simulink model "Immersion_2"  (Simulink 9.1)
settings: Solver=ode45  StartTime=0.0  StopTime=6  FixedStep=0.01  RelTol=1e-3  EnableMultiTasking=on
model workspace (MAT data in the model file):
  random_seed : num (value not decoded)
undefined symbols (not defined in the file): CafHat, CarHat, K, lam_1, lam_2, Lf, Lr, m, mu, random_seeds, Vel
libraries: simulink x2, Solver_SF x1
settings Model: Creator=xuwei  LastModifiedBy=CK12
settings DataIOCC: LimitDataPoints=on
settings OptimizationCC: ExpressionDepthLimit=2147483647
settings DebuggingCC: SolverPrmCheckMsg=warning  FcnCallInpInsideContextMsg=warning  StateNameClashWarn=warning
settings ConfigComp: CovHtmlReporting=off

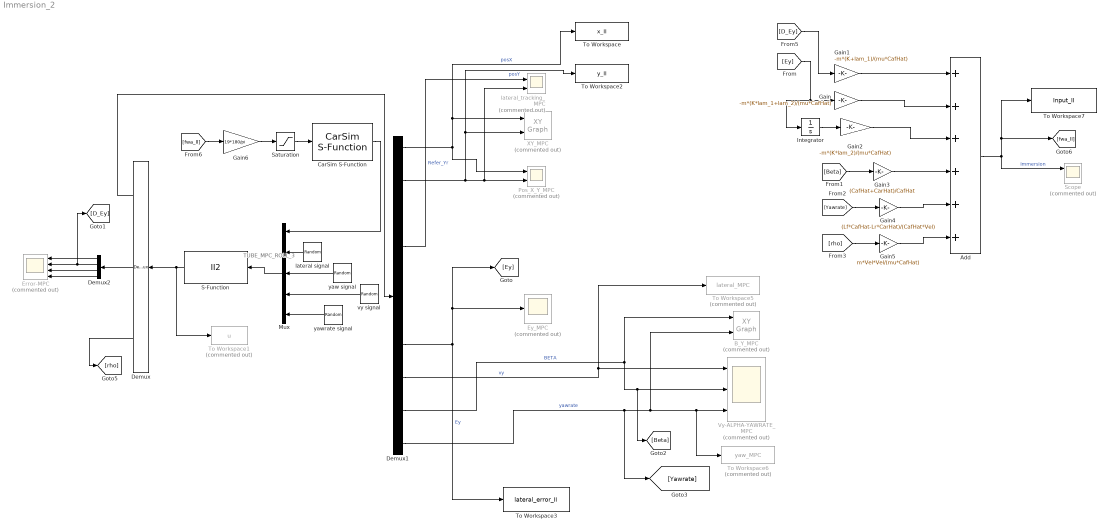
== system Immersion_2 ==
  note: TUBE_MPC_ROLL_3
  Add : Sum  Inputs=++++++
  B_Y_MPC : simulink/Sinks/XY Graph  Commented=on  xmin=-0.1  xmax=0.1  ymin=-0.9  ymax=0.9  st=-1
  CarSim S-Function : Solver_SF/CarSim S-Function  Priority=1  SIMFILE=simfile.sim  Run_RTs=off  vs_state_ind=Run  StopMode_ind=Vehicle Model
  Demux : Demux  Outputs=[10 4 1]
  Demux1 : Demux  Outputs=10
  Demux2 : Demux
  Error-MPC : Scope  Commented=on  NumInputPorts=4
  Ey_MPC : Scope  Commented=on
  Gain : Gain  Gain=-m*(K*lam_1+lam_2)/(mu*CafHat)
  Gain1 : Gain  Gain=-m*(K+lam_1)/(mu*CafHat)
  Gain2 : Gain  Gain=-m*(K*lam_2)/(mu*CafHat)
  Gain3 : Gain  Gain=(CafHat+CarHat)/CafHat
  Gain4 : Gain  Gain=(Lf*CafHat-Lr*CarHat)/(CafHat*Vel)
  Gain5 : Gain  Gain=m*Vel*Vel/(mu*CafHat)
  Gain6 : Gain  Gain=19*180/pi
  Integrator : Integrator
  Mux : Mux  Inputs=5
  Pos_X_Y_MPC : Scope  Commented=on  NumInputPorts=2
  S-Function : S-Function  FunctionName=II2  SFunctionDeploymentMode=off  EnableBusSupport=off
  Saturation : Saturate  UpperLimit=220  LowerLimit=-220
  Scope : Scope  Commented=on  NumInputPorts=2
  To Workspace : ToWorkspace  VariableName=x_II  SampleTime=-1
      settings: MaxDataPoints=data_limit
  To Workspace1 : ToWorkspace  Commented=on  VariableName=u  SaveFormat=Structure  SampleTime=-1
  To Workspace2 : ToWorkspace  VariableName=y_II  SampleTime=-1
      settings: MaxDataPoints=data_limit
  To Workspace3 : ToWorkspace  VariableName=lateral_error_II  SampleTime=-1
      settings: MaxDataPoints=data_limit
  To Workspace5 : ToWorkspace  Commented=on  VariableName=lateral_MPC  SaveFormat=Timeseries  SampleTime=-1
  To Workspace6 : ToWorkspace  Commented=on  VariableName=yaw_MPC  SaveFormat=Timeseries  SampleTime=-1
  To Workspace7 : ToWorkspace  VariableName=Input_II  SampleTime=0.05
      settings: MaxDataPoints=data_limit
  Vy-ALPHA-YAWRATE_MPC : Scope  Commented=on  NumInputPorts=3
  XY_MPC : simulink/Sinks/XY Graph  Commented=on  xmin=-10  xmax=180  ymin=-4  ymax=4  st=-1
  lateral signal : UniformRandomNumber  Minimum=-0.05  Maximum=0.05  Seed=random_seeds  SampleTime=0.1
  lateral_tracking_MPC : Scope  Commented=on  NumInputPorts=2
  vy signal : UniformRandomNumber  Minimum=-0.05  Maximum=0.05  Seed=random_seeds+1  SampleTime=0.1
  yaw signal : UniformRandomNumber  Minimum=-0.0174  Maximum=0.0174  Seed=random_seeds  SampleTime=0.1
  yawrate signal : UniformRandomNumber  Minimum=-0.0174  Maximum=0.0174  Seed=random_seeds+1  SampleTime=0.1
  wires:
  S-Function/1 -> To Workspace1/1, Demux/1
  Demux/1 -> Demux1/1
  Demux2/1 -> Error-MPC/1
  Demux2/2 -> [D_Ey], Error-MPC/2
  Demux2/3 -> Error-MPC/3
  Demux2/4 -> Error-MPC/4
  Demux/2 -> Demux2/1
  Demux1/10 -> Vy-ALPHA-YAWRATE_MPC/3, To Workspace6/1, B_Y_MPC/2, [Yawrate]  "yawrate"
  Demux1/8 -> To Workspace5/1, Vy-ALPHA-YAWRATE_MPC/1  "vy"
  Demux1/9 -> [Beta], Vy-ALPHA-YAWRATE_MPC/2, B_Y_MPC/1  "BETA"
  Demux1/4 -> lateral_tracking_MPC/1  "Refer_Yr"
  Demux1/2 -> XY_MPC/2, To Workspace2/1, Pos_X_Y_MPC/2, lateral_tracking_MPC/2  "posY"
  Demux1/1 -> Pos_X_Y_MPC/1, XY_MPC/1, To Workspace/1  "posX"
  Demux1/7 -> Ey_MPC/1, [Ey], To Workspace3/1  "Ey"
  Demux/3 -> [rho]
  [D_Ey] -> Gain1/1
  Gain4/1 -> Add/5
  [Ey] -> Integrator/1, Gain/1
  Integrator/1 -> Gain2/1
  [Yawrate] -> Gain4/1
  Add/1 -> To Workspace7/1, [fwa_II], Scope/1  "Immersion"
  Gain/1 -> Add/2
  Gain3/1 -> Add/4
  Gain1/1 -> Add/1
  [rho] -> Gain5/1
  Gain5/1 -> Add/6
  [Beta] -> Gain3/1
  Gain2/1 -> Add/3
  [fwa_II] -> Gain6/1
  Gain6/1 -> Saturation/1
  Saturation/1 -> CarSim S-Function/1
  yawrate signal/1 -> Mux/5
  CarSim S-Function/1 -> Mux/1
  lateral signal/1 -> Mux/2
  yaw signal/1 -> Mux/3
  Mux/1 -> S-Function/1
  vy signal/1 -> Mux/4
